simulink subsystem "UserInputsFOCSLHost"  (R2024b)
settings: Solver=VariableStepAuto  StartTime=0.0  StopTime=10.0  RelTol=1e-3
values from neighbouring files (symbols this model uses):
  Ts_SerialIn = 0.1    [s32k344Data.m]
libraries: svdutilitieslib x1
settings Model: Creator=The MathWorks, Inc.  LastModifiedBy=snarayan
settings RTWCC: GPUComputeCapability=3.5

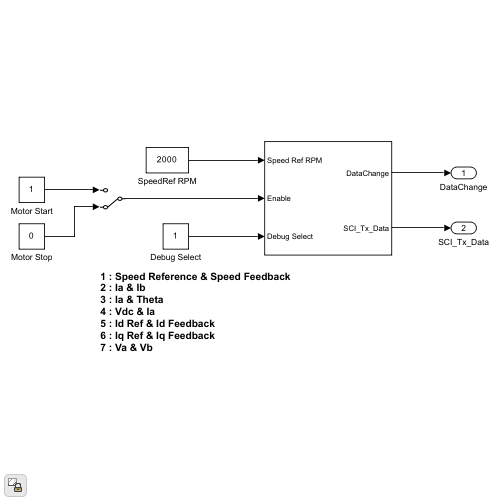
[thumbnail: Simulink's stored preview of the top-level diagram]
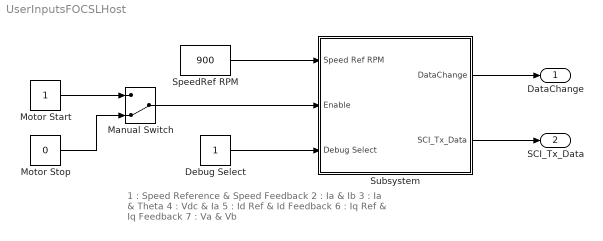
== system UserInputsFOCSLHost ==
  note: 1 : Speed Reference & Speed Feedback
      | 2 : Ia & Ib
      | 3 : Ia & Theta
      | 4 : Vdc & Ia
      | 5 : Id Ref & Id Feedback
      | 6 : Iq Ref & Iq Feedback
      | 7 : Va & Vb
  Debug Select : Constant  OutDataTypeStr=uint8  SampleTime=Ts_SerialIn
  Manual Switch : ManualSwitch  CurrentSetting=0
  Motor Start : Constant  OutDataTypeStr=uint8  SampleTime=Ts_SerialIn
  Motor Stop : Constant  Value=0  OutDataTypeStr=uint8  SampleTime=Ts_SerialIn
  SpeedRef RPM : Constant  Value=900  OutDataTypeStr=int16  SampleTime=Ts_SerialIn
  Subsystem : Subsystem
  DataChange : Outport
  SCI_Tx_Data : Outport  Port=2
  wires:
  Subsystem/1(DataChange) -> DataChange/1
  Subsystem/2(SCI_Tx_Data) -> SCI_Tx_Data/1
  SpeedRef RPM/1 -> Subsystem/1(Speed Ref RPM)
  Debug Select/1 -> Subsystem/3(Debug Select)
  Manual Switch/1 -> Subsystem/2(Enable)
  Motor Start/1 -> Manual Switch/1
  Motor Stop/1 -> Manual Switch/2

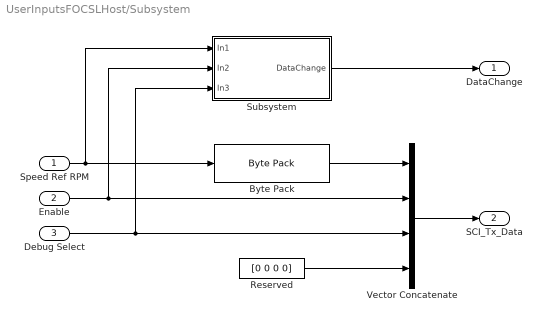
== system UserInputsFOCSLHost/Subsystem ==
  Speed Ref RPM : Inport
  Enable : Inport  Port=2
  Debug Select : Inport  Port=3
  Byte Pack : svdutilitieslib/Byte Pack  maskPackedDataType=uint8  datatypes={'int16'}  byteAlign=1  blockPlatform=arduinoert
      settings: LibrarySourceBlock=mcblib/Signal Management/Byte Pack
  Reserved : Constant  Value=[0 0 0 0]  OutDataTypeStr=uint8  SampleTime=-1
  Subsystem : Subsystem
  Vector Concatenate : Concatenate  NumInputs=4
  DataChange : Outport
  SCI_Tx_Data : Outport  Port=2
  wires:
  Vector Concatenate/1 -> SCI_Tx_Data/1
  Reserved/1 -> Vector Concatenate/4
  Byte Pack/1 -> Vector Concatenate/1
  Subsystem/1(DataChange) -> DataChange/1
  Debug Select/1 -> Vector Concatenate/3, Subsystem/3(In3)
  Enable/1 -> Vector Concatenate/2, Subsystem/2(In2)
  Speed Ref RPM/1 -> Byte Pack/1, Subsystem/1(In1)

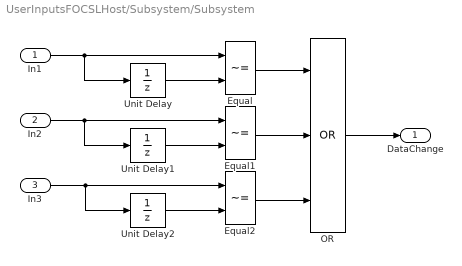
== system UserInputsFOCSLHost/Subsystem/Subsystem ==
  In1 : Inport
  In2 : Inport  Port=2
  In3 : Inport  Port=3
  Equal : RelationalOperator  Operator=~=  OutDataTypeStr=boolean  RndMeth=Simplest  InputSameDT=off
  Equal1 : RelationalOperator  Operator=~=  OutDataTypeStr=boolean  RndMeth=Simplest  InputSameDT=off
  Equal2 : RelationalOperator  Operator=~=  OutDataTypeStr=boolean  RndMeth=Simplest  InputSameDT=off
  OR : Logic  Operator=OR  Inputs=3  AllPortsSameDT=off  OutDataTypeStr=boolean
  Unit Delay : UnitDelay  SampleTime=-1  HasFrameUpgradeWarning=on
  Unit Delay1 : UnitDelay  SampleTime=-1  HasFrameUpgradeWarning=on
  Unit Delay2 : UnitDelay  SampleTime=-1  HasFrameUpgradeWarning=on
  DataChange : Outport
  wires:
  Unit Delay2/1 -> Equal2/2
  OR/1 -> DataChange/1
  Equal2/1 -> OR/3
  Unit Delay/1 -> Equal/2
  Equal1/1 -> OR/2
  Equal/1 -> OR/1
  Unit Delay1/1 -> Equal1/2
  In3/1 -> Unit Delay2/1, Equal2/1
  In1/1 -> Equal/1, Unit Delay/1
  In2/1 -> Equal1/1, Unit Delay1/1
